simulink model "gmStateSpaceHDL_uz_inverter_3ph"  (R2021b)
settings: Solver=FixedStepDiscrete  StartTime=0.0  StopTime=0.6  FixedStep=Auto  RelTol=1e-3
InitFcn:
  | load('C:\Users\valen\Documents\repos\UZ\ultrazohm_sw\ip_cores\uz_inverter_3ph\sschdl\uz_inverter_3ph\stateSpaceParameters.mat');
values from neighbouring files (symbols this model uses):
  stateSpaceParameters_1 =     [stateSpaceParameters.mat]
undefined symbols (not defined in the file or in its folder): g1, g2, g3, g4, g5, g6, i_a, i_b, i_c, pslcontrol, ts
libraries: hdlssclib x2
settings Model: Creator=LENOVO  LastModifiedBy=valen
settings SolverCC: AlgebraicLoopSolver=TrustRegion
settings DataIOCC: LimitDataPoints=on  SaveOutput=off  SaveTime=off
settings OptimizationCC: BlockReduction=off  ConditionallyExecuteInputs=off  DefaultParameterBehavior=Inlined  InheritOutputTypeSmallerThanSingle=on  LifeSpan=inf
settings DebuggingCC: AlgebraicLoopMsg=error  SingleTaskRateTransMsg=error  AllowSymbolicDim=off  StrictBusMsg=ErrorOnBusTreatedAsVector  SFUnexpectedBacktrackingDiag=warning  SFNoUnconditionalDefaultTransitionDiag=warning  SFExecutionAtInitializationDiag=none  SFMachineParentedDataDiag=warning  ArithmeticOperatorsInVariantConditions=warning
settings HardwareCC: ProdBitPerPointer=32  ProdBitPerSizeT=32  ProdBitPerPtrDiffT=32  ProdLargestAtomicFloat=None  ProdIntDivRoundTo=Undefined  ProdEndianess=Unspecified  ProdWordSize=32  ProdHWDeviceType=ASIC/FPGA->ASIC/FPGA  ProdEqTarget=off
settings SFSimCC: SimUseLocalCustomCode=off  CustomCodeUndefinedFunction=UseInterfaceOnly
settings RTWCC: RTWUseLocalCustomCode=off
settings CodeAppCC: StateflowObjectComments=on
settings GRTTargetCC: TargetLangStandard=C89/C90 (ANSI)
settings ConfigComp: CovScope=ReferencedModels  CovMetricSettings=dw  CovSaveCumulativeToWorkspaceVar=on  CovSaveSingleToWorkspaceVar=on  CovExternalEMLEnable=off  CovSFcnEnable=off

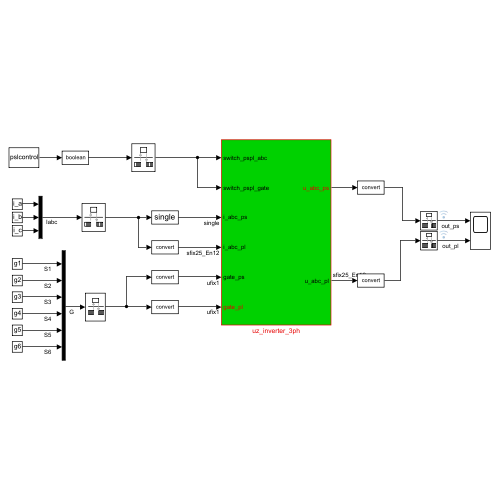
[thumbnail: Simulink's stored preview of the top-level diagram]
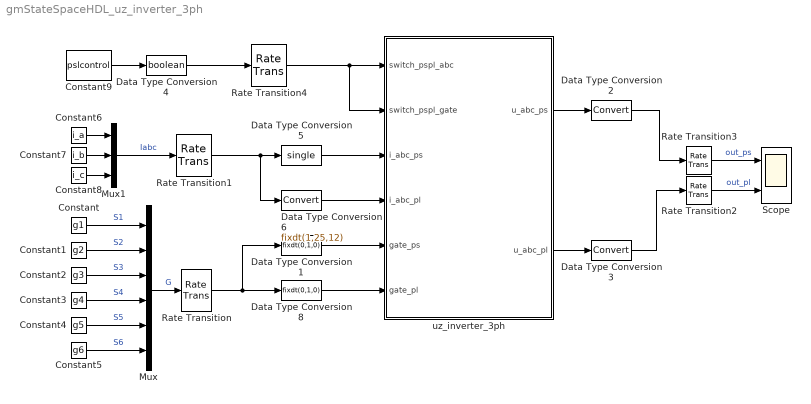
== system gmStateSpaceHDL_uz_inverter_3ph ==
  Constant : Constant  Value=g1  SampleTime=ts
  Constant1 : Constant  Value=g2  SampleTime=ts
  Constant2 : Constant  Value=g3  SampleTime=ts
  Constant3 : Constant  Value=g4  SampleTime=ts
  Constant4 : Constant  Value=g5  SampleTime=ts
  Constant5 : Constant  Value=g6  SampleTime=ts
  Constant6 : Constant  Value=i_a  SampleTime=ts
  Constant7 : Constant  Value=i_b  SampleTime=ts
  Constant8 : Constant  Value=i_c  SampleTime=ts
  Constant9 : Constant  Value=pslcontrol
  Data Type Conversion1 : DataTypeConversion  OutMin=0  OutMax=1  OutDataTypeStr=fixdt(0,1,0)  RndMeth=Nearest
  Data Type Conversion2 : DataTypeConversion
  Data Type Conversion3 : DataTypeConversion
  Data Type Conversion4 : DataTypeConversion  OutDataTypeStr=boolean
  Data Type Conversion5 : DataTypeConversion  OutDataTypeStr=single  RndMeth=Nearest
  Data Type Conversion6 : DataTypeConversion  OutDataTypeStr=fixdt(1,25,12)  RndMeth=Nearest
  Data Type Conversion8 : DataTypeConversion  OutMin=0  OutMax=1  OutDataTypeStr=fixdt(0,1,0)  RndMeth=Nearest
  Mux : Mux  Inputs=6
  Mux1 : Mux  Inputs=3
  Rate Transition{,1..4} (5 alike) : RateTransition  OutPortSampleTime=ts
  Scope : Scope  NumInputPorts=2
  uz_inverter_3ph : Subsystem
  wires:
  uz_inverter_3ph/1(u_abc_ps) -> Data Type Conversion2/1
  uz_inverter_3ph/2(u_abc_pl) -> Data Type Conversion3/1
  Data Type Conversion3/1 -> Rate Transition2/1
  Data Type Conversion2/1 -> Rate Transition3/1
  Rate Transition3/1 -> Scope/1  "out_ps"
  Rate Transition2/1 -> Scope/2  "out_pl"
  Data Type Conversion4/1 -> Rate Transition4/1
  Rate Transition4/1 -> uz_inverter_3ph/1(switch_pspl_abc), uz_inverter_3ph/2(switch_pspl_gate)
  Constant9/1 -> Data Type Conversion4/1
  Constant2/1 -> Mux/3  "S3"
  Constant4/1 -> Mux/5  "S5"
  Constant5/1 -> Mux/6  "S6"
  Constant3/1 -> Mux/4  "S4"
  Mux1/1 -> Rate Transition1/1  "Iabc"
  Mux/1 -> Rate Transition/1  "G"
  Constant8/1 -> Mux1/3
  Constant6/1 -> Mux1/1
  Constant1/1 -> Mux/2  "S2"
  Constant7/1 -> Mux1/2
  Constant/1 -> Mux/1  "S1"
  Rate Transition1/1 -> Data Type Conversion5/1, Data Type Conversion6/1
  Data Type Conversion6/1 -> uz_inverter_3ph/4(i_abc_pl)
  Data Type Conversion8/1 -> uz_inverter_3ph/6(gate_pl)
  Rate Transition/1 -> Data Type Conversion8/1, Data Type Conversion1/1
  Data Type Conversion1/1 -> uz_inverter_3ph/5(gate_ps)
  Data Type Conversion5/1 -> uz_inverter_3ph/3(i_abc_ps)

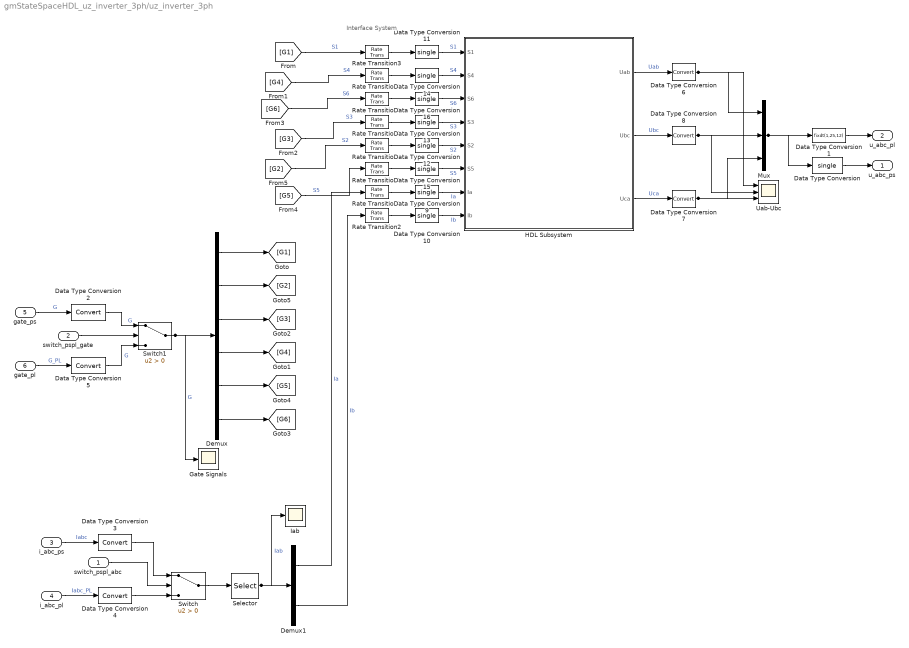
== system gmStateSpaceHDL_uz_inverter_3ph/uz_inverter_3ph ==
  note: Interface System
  switch_pspl_abc : Inport
  switch_pspl_gate : Inport  Port=2
  i_abc_ps : Inport  Port=3  OutDataTypeStr=single
  i_abc_pl : Inport  Port=4  OutDataTypeStr=fixdt(1,25,12)
  gate_ps : Inport  Port=5  OutDataTypeStr=fixdt(0,1,0)  LockScale=on
  gate_pl : Inport  Port=6  OutDataTypeStr=fixdt(0,1,0)
  Data Type Conversion{,9..16} (9 alike) : DataTypeConversion  OutDataTypeStr=single  RndMeth=Nearest
  Data Type Conversion1 : DataTypeConversion  OutDataTypeStr=fixdt(1,25,12)  RndMeth=Nearest
  Data Type Conversion{2..8} (7 alike) : DataTypeConversion  RndMeth=Nearest
  Demux : Demux  Outputs=6
  Demux1 : Demux  Outputs=2
  Gate Signals : Scope
  HDL Subsystem : Subsystem
  Iab : Scope
  Mux : Mux  Inputs=3
  Rate Transition{1..8} (8 alike) : RateTransition  OutPortSampleTime=5e-07
  Selector : Selector  InputPortWidth=3  IndexOptions=Index vector (dialog)  Indices=[1 2]  OutputSizes=1
  Switch : Switch  Criteria=u2 > Threshold
  Switch1 : Switch  Criteria=u2 > Threshold
  Uab-Ubc : Scope  NumInputPorts=3
  u_abc_ps : Outport
  u_abc_pl : Outport  Port=2  OutDataTypeStr=fixdt(1,25,12)
  wires:
  Data Type Conversion8/1 -> Mux/2, Uab-Ubc/2
  Data Type Conversion6/1 -> Mux/1, Uab-Ubc/1
  Rate Transition1/1 -> Data Type Conversion9/1
  Data Type Conversion7/1 -> Uab-Ubc/3, Mux/3
  switch_pspl_gate/1 -> Switch1/2
  Data Type Conversion2/1 -> Switch1/1  "G"
  Switch1/1 -> Demux/1, Gate Signals/1  "G"
  Data Type Conversion/1 -> u_abc_ps/1
  Data Type Conversion1/1 -> u_abc_pl/1
  Data Type Conversion11/1 -> HDL Subsystem/1(S1)  "S1"
  Mux/1 -> Data Type Conversion/1, Data Type Conversion1/1
  Data Type Conversion5/1 -> Switch1/3  "G"
  Rate Transition3/1 -> Data Type Conversion11/1
  switch_pspl_abc/1 -> Switch/2
  Rate Transition5/1 -> Data Type Conversion13/1
  Data Type Conversion13/1 -> HDL Subsystem/4(S3)  "S3"
  Data Type Conversion12/1 -> HDL Subsystem/5(S2)  "S2"
  Rate Transition8/1 -> Data Type Conversion16/1
  Data Type Conversion15/1 -> HDL Subsystem/6(S5)  "S5"
  Data Type Conversion9/1 -> HDL Subsystem/7(Ia)  "Ia"
  Data Type Conversion10/1 -> HDL Subsystem/8(Ib)  "Ib"
  Data Type Conversion16/1 -> HDL Subsystem/3(S6)  "S6"
  Data Type Conversion14/1 -> HDL Subsystem/2(S4)  "S4"
  Rate Transition7/1 -> Data Type Conversion15/1
  Rate Transition6/1 -> Data Type Conversion14/1
  Rate Transition4/1 -> Data Type Conversion12/1
  Rate Transition2/1 -> Data Type Conversion10/1
  gate_pl/1 -> Data Type Conversion5/1  "G_PL"
  gate_ps/1 -> Data Type Conversion2/1  "G"
  Demux/5 -> [G5]
  Demux/2 -> [G2]
  Demux/1 -> [G1]
  Demux/3 -> [G3]
  Demux/4 -> [G4]
  Demux/6 -> [G6]
  Data Type Conversion4/1 -> Switch/3
  Data Type Conversion3/1 -> Switch/1
  i_abc_ps/1 -> Data Type Conversion3/1  "Iabc"
  i_abc_pl/1 -> Data Type Conversion4/1  "Iabc_PL"
  Switch/1 -> Selector/1
  Selector/1 -> Demux1/1, Iab/1  "Iab"
  [G3] -> Rate Transition5/1  "S3"
  [G1] -> Rate Transition3/1  "S1"
  [G2] -> Rate Transition4/1  "S2"
  [G4] -> Rate Transition6/1  "S4"
  [G5] -> Rate Transition7/1  "S5"
  [G6] -> Rate Transition8/1  "S6"
  HDL Subsystem/3(Uca) -> Data Type Conversion7/1  "Uca"
  HDL Subsystem/2(Ubc) -> Data Type Conversion8/1  "Ubc"
  HDL Subsystem/1(Uab) -> Data Type Conversion6/1  "Uab"
  Demux1/2 -> Rate Transition2/1  "Ib"
  Demux1/1 -> Rate Transition1/1  "Ia"

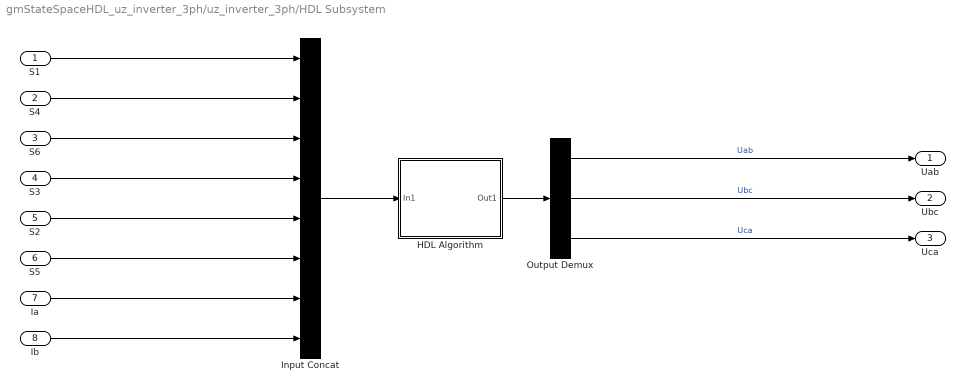
== system gmStateSpaceHDL_uz_inverter_3ph/uz_inverter_3ph/HDL Subsystem ==
  S1 : Inport
  S4 : Inport  Port=2
  S6 : Inport  Port=3
  S3 : Inport  Port=4
  S2 : Inport  Port=5
  S5 : Inport  Port=6
  Ia : Inport  Port=7
  Ib : Inport  Port=8
  HDL Algorithm : Subsystem
  Input Concat : Concatenate  NumInputs=8
  Output Demux : Demux  Outputs=3
  Uab : Outport
  Ubc : Outport  Port=2
  Uca : Outport  Port=3
  wires:
  HDL Algorithm/1(Out1) -> Output Demux/1
  S3/1 -> Input Concat/4
  S6/1 -> Input Concat/3
  S5/1 -> Input Concat/6
  Input Concat/1 -> HDL Algorithm/1(In1)
  S1/1 -> Input Concat/1
  S2/1 -> Input Concat/5
  Ia/1 -> Input Concat/7
  Output Demux/1 -> Uab/1  "Uab"
  Output Demux/3 -> Uca/1  "Uca"
  S4/1 -> Input Concat/2
  Output Demux/2 -> Ubc/1  "Ubc"
  Ib/1 -> Input Concat/8

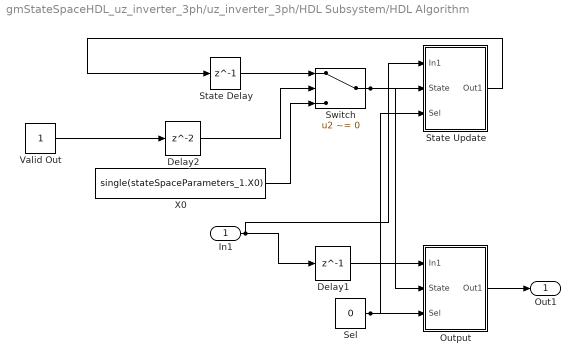
== system gmStateSpaceHDL_uz_inverter_3ph/uz_inverter_3ph/HDL Subsystem/HDL Algorithm ==
  In1 : Inport
  Delay1 : Delay  DelayLength=1
  Delay2 : Delay
  Output : Subsystem
  Sel : Constant  Value=0  OutDataTypeStr=uint32  SampleTime=5e-07
  State Delay : Delay  DelayLength=1  InitialCondition=single(stateSpaceParameters_1.X0)
  State Update : Subsystem
  Switch : Switch  Criteria=u2 ~= 0
  Valid Out : Constant  OutDataTypeStr=boolean  SampleTime=5e-07
  X0 : Constant  Value=single(stateSpaceParameters_1.X0)  SampleTime=5e-07
  Out1 : Outport  VectorParamsAs1DForOutWhenUnconnected=off
  wires:
  X0/1 -> Switch/3
  Valid Out/1 -> Delay2/1
  Delay2/1 -> Switch/2
  Output/1(Out1) -> Out1/1
  Switch/1 -> State Update/2(State), Output/2(State)
  State Delay/1 -> Switch/1
  State Update/1(Out1) -> State Delay/1
  Delay1/1 -> Output/1(In1)
  In1/1 -> State Update/1(In1), Delay1/1
  Sel/1 -> State Update/3(Sel), Output/3(Sel)

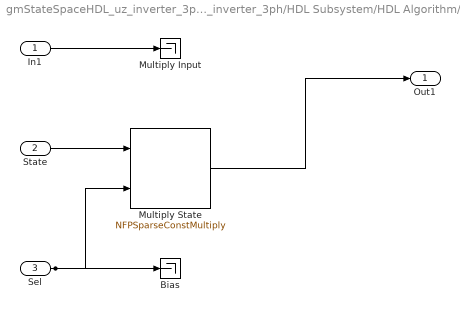
== system gmStateSpaceHDL_uz_inverter_3ph/uz_inverter_3ph/HDL Subsystem/HDL Algorithm/Output ==
  In1 : Inport
  State : Inport  Port=2
  Sel : Inport  Port=3
  Bias : Terminator
  Multiply Input : Terminator
  Multiply State : hdlssclib/NFPSparseConstMultiply  constMatrix=single(stateSpaceParameters_1.Cd)
      settings: SourceProductBaseCode=SL
  Out1 : Outport  VectorParamsAs1DForOutWhenUnconnected=off
  wires:
  State/1 -> Multiply State/1
  In1/1 -> Multiply Input/1
  Sel/1 -> Bias/1, Multiply State/2
  Multiply State/1 -> Out1/1

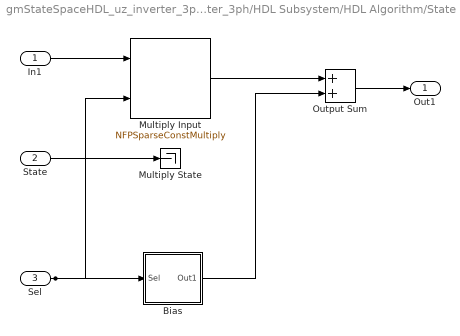
== system gmStateSpaceHDL_uz_inverter_3ph/uz_inverter_3ph/HDL Subsystem/HDL Algorithm/State Update ==
  In1 : Inport
  State : Inport  Port=2
  Sel : Inport  Port=3
  Bias : Subsystem
  Multiply Input : hdlssclib/NFPSparseConstMultiply  constMatrix=single(stateSpaceParameters_1.Bd)
      settings: SourceProductBaseCode=SL
  Multiply State : Terminator
  Output Sum : Sum
  Out1 : Outport  OutDataTypeStr=single  VectorParamsAs1DForOutWhenUnconnected=off
  wires:
  State/1 -> Multiply State/1
  In1/1 -> Multiply Input/1
  Sel/1 -> Bias/1(Sel), Multiply Input/2
  Output Sum/1 -> Out1/1
  Multiply Input/1 -> Output Sum/1
  Bias/1(Out1) -> Output Sum/2

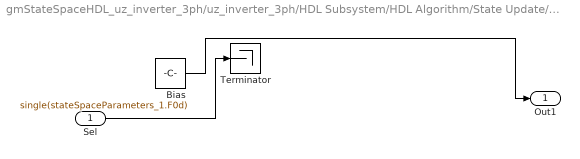
== system gmStateSpaceHDL_uz_inverter_3ph/uz_inverter_3ph/HDL Subsystem/HDL Algorithm/State Update/Bias ==
  Sel : Inport
  Bias : Constant  Value=single(stateSpaceParameters_1.F0d)  SampleTime=5e-07
  Terminator : Terminator
  Out1 : Outport  VectorParamsAs1DForOutWhenUnconnected=off
  wires:
  Sel/1 -> Terminator/1
  Bias/1 -> Out1/1
